simulink model "Optimal_b"  (R2016b)
settings: Solver=FixedStepAuto  StartTime=0.0  StopTime=1.5  FixedStep=0.01  RelTol=1e-3
values from neighbouring files (symbols this model uses):
  dt = 0.01    [Game_Space.m]    (also in parameters.m; vec_s1.mat)
  K = 0.2*sgn    [parameters.m]    (also in vec_s1.mat = 0.2)
  K_dth = 0.2*sgn    [parameters.m]    (also in vec_s1.mat = 0.05)
  m = max_m(i)*jj(j)    [Proj_2.m]
  M_d = 200*sgn    [parameters.m]    (also in vec_s1.mat = 200)
  mu = mu^-1    (= 2)    [Game_Space.m]    (also in Proj_2.m = mu_r(i))
  rho_u = rho_v/mu_r(i)    [Proj_2.m]    (also in parameters.m = 75; vec_s1.mat = 75)
  t_go = tf-t    [Game_Space.m]    (also in Proj_2.m = t_go_m(i))
  T_m = 120    [parameters.m]    (also in vec_s1.mat)
  tau = 0.05    [parameters.m]    (also in vec_s1.mat)
settings Model: Creator=Daniel  LastModifiedBy=Daniel

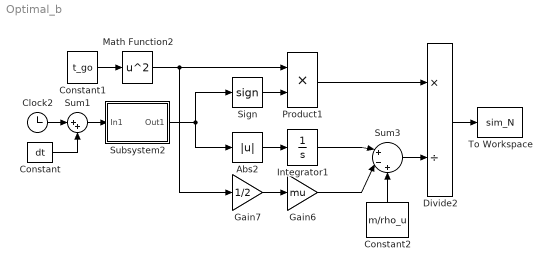
== system Optimal_b ==
  Abs2 : Abs
  Clock2 : Clock
  Constant : Constant  Value=dt
  Constant1 : Constant  Value=t_go
  Constant2 : Constant  Value=m/rho_u
  Divide2 : Product  Inputs=*/
  Gain6 : Gain  Gain=mu
  Gain7 : Gain  Gain=1/2
  Integrator1 : Integrator
  Math Function2 : Math  Operator=square  SaturateOnIntegerOverflow=on
  Product1 : Product
  Sign : Signum
  Subsystem2 : Subsystem
      mask Display: image('Gm_s_F.png');
  Sum1 : Sum  Inputs=|++
  Sum3 : Sum  Inputs=|+-+
  To Workspace : ToWorkspace  VariableName=sim_N  SaveFormat=Timeseries  SampleTime=-1
  wires:
  Subsystem2/1(Out1) -> Abs2/1, Sign/1
  Sum1/1 -> Subsystem2/1(In1)
  Math Function2/1 -> Gain7/1, Product1/1
  Abs2/1 -> Integrator1/1
  Integrator1/1 -> Sum3/1
  Product1/1 -> Divide2/1
  Sign/1 -> Product1/2
  Gain6/1 -> Sum3/2
  Gain7/1 -> Gain6/1
  Sum3/1 -> Divide2/2
  Divide2/1 -> To Workspace/1
  Clock2/1 -> Sum1/1
  Constant/1 -> Sum1/2
  Constant1/1 -> Math Function2/1
  Constant2/1 -> Sum3/3

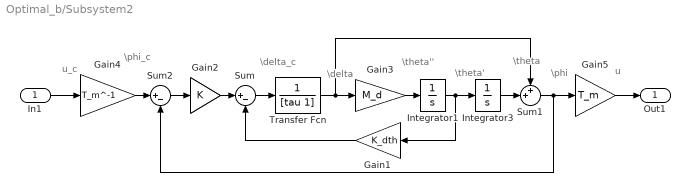
== system Optimal_b/Subsystem2 ==
  note: u_c
  note: u
  note: \phi
  note: \phi_c
  note: \delta_c
  note: \delta
  note: \theta
  note: \theta''
  note: \theta'
  In1 : Inport
  Gain1 : Gain  Gain=K_dth
  Gain2 : Gain  Gain=K
  Gain3 : Gain  Gain=M_d
  Gain4 : Gain  Gain=T_m^-1
  Gain5 : Gain  Gain=T_m
  Integrator1 : Integrator
  Integrator3 : Integrator
  Sum : Sum  Inputs=|+-
  Sum1 : Sum  Inputs=++|
  Sum2 : Sum  Inputs=|+-
  Transfer Fcn : TransferFcn  Denominator=[tau 1]
  Out1 : Outport
  wires:
  Transfer Fcn/1 -> Gain3/1, Sum1/1
  Gain2/1 -> Sum/1
  Integrator3/1 -> Sum1/2
  Gain4/1 -> Sum2/1
  Gain5/1 -> Out1/1
  Sum2/1 -> Gain2/1
  In1/1 -> Gain4/1
  Gain1/1 -> Sum/2
  Sum/1 -> Transfer Fcn/1
  Sum1/1 -> Gain5/1, Sum2/2
  Integrator1/1 -> Gain1/1, Integrator3/1
  Gain3/1 -> Integrator1/1
